simulink model "MagnetoShield_PolePlacement_Simulation_TEXT"  (R2019a)
settings: Solver=VariableStepAuto  StartTime=0.0  StopTime=15  RelTol=1e-3
undefined symbols (not defined in the file): A, B, C, DiscIntNeverNeededParam, i0, K, L, sigbuilder_block, Ts, u0, y0
libraries: simulink x2
settings Model: Creator=jakub  LastModifiedBy=jakub

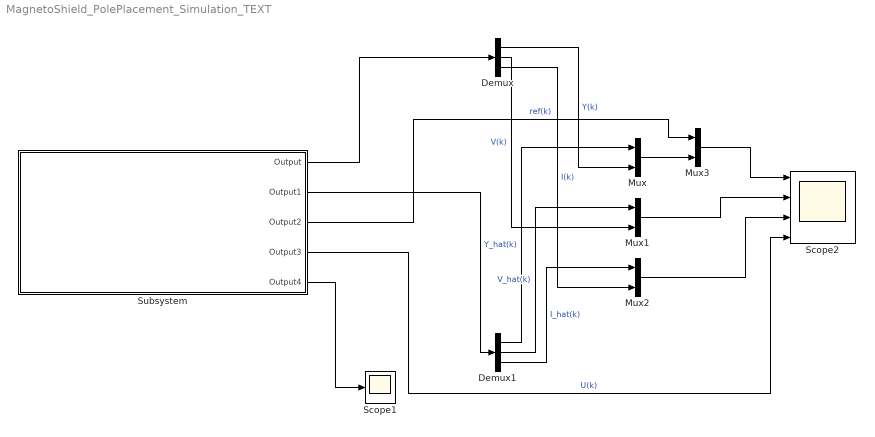
== system MagnetoShield_PolePlacement_Simulation_TEXT ==
  Demux : Demux  Outputs=3
  Demux1 : Demux  Outputs=3
  Mux{,1..3} (4 alike) : Mux  Inputs=2
  Scope1 : Scope
  Scope2 : Scope  NumInputPorts=4
  Subsystem : Subsystem
  wires:
  Mux/1 -> Mux3/2
  Mux2/1 -> Scope2/3
  Demux1/2 -> Mux1/1  "V_hat(k)"
  Demux1/3 -> Mux2/1  "I_hat(k)"
  Demux/1 -> Mux/2  "Y(k)"
  Mux1/1 -> Scope2/2
  Demux/3 -> Mux2/2  "I(k)"
  Demux1/1 -> Mux/1  "Y_hat(k)"
  Demux/2 -> Mux1/2  "V(k)"
  Subsystem/5(Output4) -> Scope1/1
  Subsystem/1(Output) -> Demux/1
  Subsystem/3(Output2) -> Mux3/1  "ref(k)"
  Mux3/1 -> Scope2/1
  Subsystem/4(Output3) -> Scope2/4  "U(k)"
  Subsystem/2(Output1) -> Demux1/1

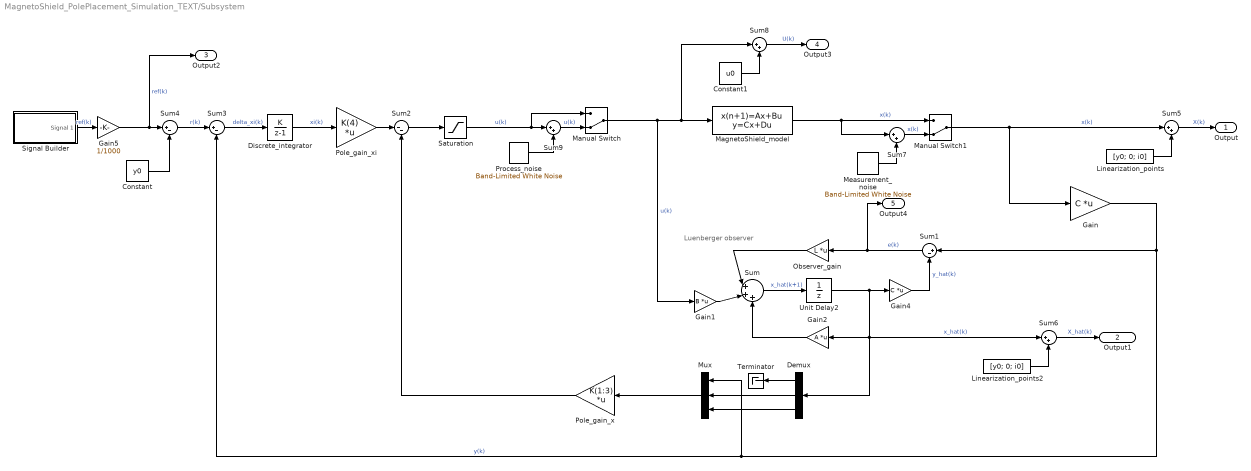
== system MagnetoShield_PolePlacement_Simulation_TEXT/Subsystem ==
  note: Luenberger observer
  Constant : Constant  Value=y0
  Constant1 : Constant  Value=u0
  Demux : Demux  Outputs=3
  Discrete_integrator : DiscreteIntegrator  IntegratorMethod=Accumulation: Forward Euler  SampleTime=Ts  LimitOutput=on  UpperSaturationLimit=1  LowerSaturationLimit=-1  ICPrevOutput=DiscIntNeverNeededParam  ICPrevScaledInput=DiscIntNeverNeededParam
  Gain : Gain  Gain=C  Multiplication=Matrix(K*u)
  Gain1 : Gain  Gain=B  Multiplication=Matrix(K*u)
  Gain2 : Gain  Gain=A  Multiplication=Matrix(K*u)
  Gain4 : Gain  Gain=C  Multiplication=Matrix(K*u)
  Gain5 : Gain  Gain=1/1000
  Linearization_points : Constant  Value=[y0; 0; i0]
  Linearization_points2 : Constant  Value=[y0; 0; i0]
  MagnetoShield_model : DiscreteStateSpace  A=A  B=B  C=[1 0 0;0 1 0;0 0 1]  D=[0;0;0]  InitialCondition=[0.017-y0;0;0-i0]  SampleTime=Ts
  Manual Switch : ManualSwitch  CurrentSetting=0
  Manual Switch1 : ManualSwitch  CurrentSetting=0
  Measurement_noise : simulink/Sources/Band-Limited White Noise  Cov=[(6*10^(-7))^2]  Ts=2*Ts  seed=[23341]
  Mux : Mux  Inputs=3
  Observer_gain : Gain  Gain=L  Multiplication=Matrix(K*u)
  Pole_gain_x : Gain  Gain=K(1:3)  Multiplication=Matrix(K*u)
  Pole_gain_xi : Gain  Gain=K(4)  Multiplication=Matrix(K*u)
  Process_noise : simulink/Sources/Band-Limited White Noise  Cov=[(2*10^(-3))^2]  Ts=2*Ts  seed=[23341]
  Saturation : Saturate  UpperLimit=10-u0  LowerLimit=0-u0
  Signal Builder : Subsystem  Tag=STV Subsys  LoadFcn=sigbuilder_block('load');  StartFcn=sigbuilder_block('start');  StopFcn=sigbuilder_block('stop');  ClipboardFcn=sigbuilder_block('clipboard');  mask(Sigbuilder block){tuvar=[0:10]}
      mask help: Simulink:masks:SigbuilderBlock_MD
      mask init:
      | if ~strcmp(get_param(bdroot(gcbh),'SimulationStatus'),'stopped') tuvar = sigbuilder_block('maskInit'); end
      settings: CopyFcn=sigbuilder_block('copy');  DeleteFcn=sigbuilder_block('delete');  ModelCloseFcn=sigbuilder_block('modelClose');  PreSaveFcn=sigbuilder_block('preSave');  PauseFcn=sigbuilder_block('pause');  ContinueFcn=sigbuilder_block('continue');  NameChangeFcn=sigbuilder_block('namechange');  OpenFcn=sigbuilder_block('open',[434.4 169.8 550.8 400.2 ]);  CloseFcn=sigbuilder_block('close');
      mask Display: plot(0, 0, 100, 100,[2, 2, 32, 32, 2], [68, 8, 8, 68, 68],[32, 2], [38, 38], [32, 19, 2],[53, 60, 44], [32, 17, 17, 2],[16, 16, 31, 31]);txt = getActiveGroup(gcbh);text(2, 100, txt,'verticalAlignment', 'top');
  Sum : Sum  Inputs=|+++
  Sum1 : Sum  Inputs=|+-
  Sum2 : Sum  Inputs=|--
  Sum3 : Sum  Inputs=|+-
  Sum4 : Sum  Inputs=|+-
  Sum{5..9} (5 alike) : Sum  Inputs=|++
  Terminator : Terminator
  Unit Delay2 : UnitDelay  InitialCondition=[0.017-y0;0;0-i0]  SampleTime=-1  HasFrameUpgradeWarning=on
  Output : Outport
  Output1 : Outport  Port=2
  Output2 : Outport  Port=3
  Output3 : Outport  Port=4
  Output4 : Outport  Port=5
  wires:
  Constant/1 -> Sum4/2
  Sum1/1 -> Output4/1, Observer_gain/1  "e(k)"
  Sum6/1 -> Output1/1  "X_hat(k)"
  Sum3/1 -> Discrete_integrator/1  "delta_xi(k)"
  Gain2/1 -> Sum/3
  Pole_gain_xi/1 -> Sum2/1
  Gain5/1 -> Output2/1, Sum4/1  "ref(k)"
  Gain4/1 -> Sum1/2  "y_hat(k)"
  Linearization_points2/1 -> Sum6/2
  Pole_gain_x/1 -> Sum2/2
  Discrete_integrator/1 -> Pole_gain_xi/1  "xi(k)"
  Sum8/1 -> Output3/1  "U(k)"
  Observer_gain/1 -> Sum/1
  Gain1/1 -> Sum/2
  Sum5/1 -> Output/1  "X(k)"
  Sum/1 -> Unit Delay2/1  "x_hat(k+1)"
  Gain/1 -> Sum1/1, Sum3/2, Mux/1  "y(k)"
  Linearization_points/1 -> Sum5/2
  Sum4/1 -> Sum3/1  "r(k)"
  Constant1/1 -> Sum8/2
  Signal Builder/1(Signal 1) -> Gain5/1  "ref(k)"
  Manual Switch1/1 -> Gain/1, Sum5/1  "x(k)"
  Manual Switch/1 -> Gain1/1, Sum8/1, MagnetoShield_model/1  "u(k)"
  Sum2/1 -> Saturation/1
  MagnetoShield_model/1 -> Manual Switch1/1, Sum7/1  "x(k)"
  Saturation/1 -> Sum9/1, Manual Switch/1  "u(k)"
  Sum9/1 -> Manual Switch/2  "u(k)"
  Process_noise/1 -> Sum9/2
  Sum7/1 -> Manual Switch1/2  "x(k)"
  Measurement_noise/1 -> Sum7/2
  Demux/2 -> Mux/2
  Demux/3 -> Mux/3
  Mux/1 -> Pole_gain_x/1
  Unit Delay2/1 -> Gain4/1, Demux/1, Gain2/1, Sum6/1  "x_hat(k)"
  Demux/1 -> Terminator/1

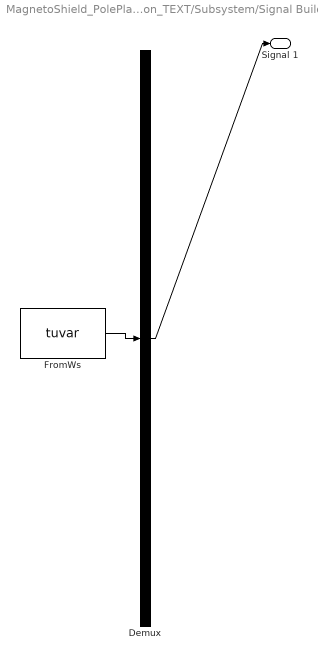
== system MagnetoShield_PolePlacement_Simulation_TEXT/Subsystem/Signal Builder ==
  Demux : Demux  Tag=STV Demux  Outputs=1
  FromWs : FromWorkspace  Tag=STV FromWs  VariableName=tuvar  SampleTime=0
      SigBuilderData=|
      | common.afterFinalStr = 'Extrapolate'
      | common.sampleTime = 0
      | dataSet.timeRange = [0 15]
      | dataSet.name = 'Group 1'
      | sbobj.Groups.Name = 'Group 1'
      | sbobj.Groups.Signals.Name = 'Signal 1'
      | sbobj.Groups.Signals.XData = [0 2 2 4 4 6 6 8 10 12 14 14 15]
      | sbobj.Groups.Signals.YData = [15.5 15.5 14 14 12.5 12.5 14.5 14.5 17 12 14.5 17 17]
      | sbobj.Groups.TimeRange = [0 15]
  Signal 1 : Outport  Tag=STV Outport
  wires:
  FromWs/1 -> Demux/1
  Demux/1 -> Signal 1/1
